simulink model "ShipMPC"  (R2020a)
settings: Solver=VariableStepAuto  StartTime=0.0  StopTime=100  RelTol=1e-3
values from neighbouring files (symbols this model uses):
  tau_wave_amp = 0    [MPCobject.m]
  tau_wave_freq = 0    [MPCobject.m]
  Vc = 0    [MPCobject.m]
  Vref = 0.1    [MPCobject.m]
libraries: mpclib x1
settings Model: Creator=ahaseltalab  LastModifiedBy=localadmin
settings DataIOCC: ReturnWorkspaceOutputs=off
settings DebuggingCC: ArithmeticOperatorsInVariantConditions=warning
settings SFSimCC: SimUseLocalCustomCode=off  CustomCodeUndefinedFunction=UseInterfaceOnly
settings RTWCC: RTWUseLocalCustomCode=off
settings CodeAppCC: StateflowObjectComments=on

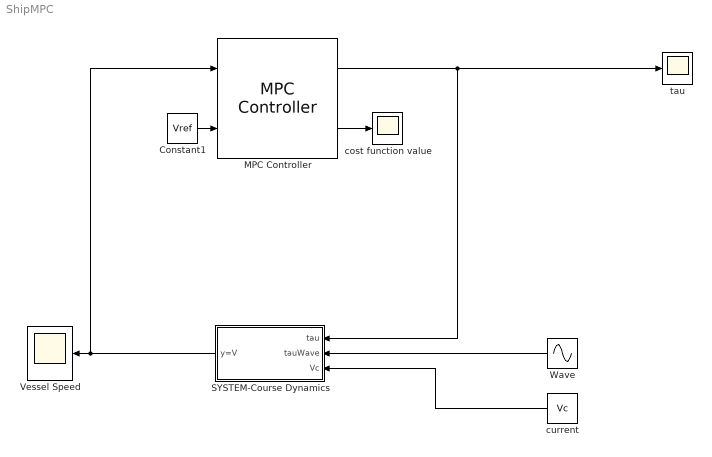
== system ShipMPC ==
  " Wave" : Sin  Amplitude=tau_wave_amp  Frequency=tau_wave_freq  SampleTime=0
  Constant1 : Constant  Value=Vref
  MPC Controller : mpclib/MPC Controller  SCDEnableBlockLinearizationSpecification=on  mpcobj=MPCobj  is_multiple=0  enable_value=0  return_u0=off  updateMPCinCallerWorkspace=on  md_inport=off  mv_inport=off  uref_inport=off  return_cost=on  return_mvseq=off  return_qpstatus=off  return_xseq=off  return_state=off  return_ovseq=off  state_inport=off  umin_inport=off  umax_inport=off  ymin_inport=off  ymax_inport=off  cc_inport=off  ywt_inport=off  uwt_inport=off  duwt_inport=off  rhoeps_inport=off  pm_inport=off  MaximumP=10  HorizonChoice=FixedHorizon  n_ts=1  n_p=20  n_mv=1  n_md=0  n_ud=0  n_mo=1  n_uo=0  BlockDataType=double  SampleTimeInherited=off  switch_inport=off
  SYSTEM-Course Dynamics : Subsystem
  Vessel Speed : Scope
  cost function value : Scope
  current : Constant  Value=Vc
  tau : Scope
  wires:
  MPC Controller/1 -> tau/1, SYSTEM-Course Dynamics/1(tau)
  MPC Controller/2 -> cost function value/1
  Constant1/1 -> MPC Controller/2
  SYSTEM-Course Dynamics/1(y=V) -> MPC Controller/1, Vessel Speed/1
  " Wave"/1 -> SYSTEM-Course Dynamics/2(tauWave)
  current/1 -> SYSTEM-Course Dynamics/3(Vc)

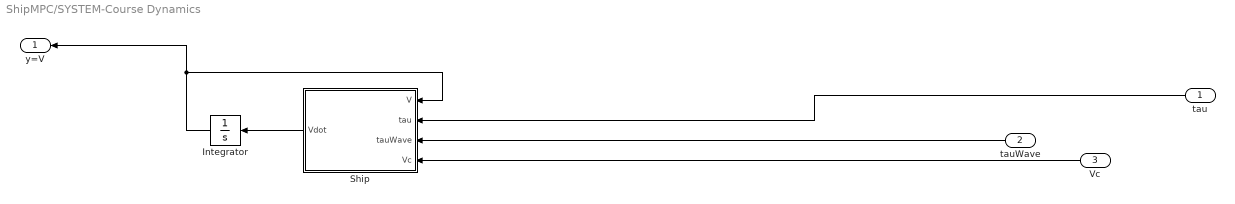
== system ShipMPC/SYSTEM-Course Dynamics ==
  tau : Inport
  tauWave : Inport  Port=2
  Vc : Inport  Port=3
  Integrator : Integrator
  Ship : MATLAB Function  TreatAsAtomicUnit=on
  y=V : Outport
  wires:
  Vc/1 -> Ship/4(Vc)
  tauWave/1 -> Ship/3(tauWave)
  tau/1 -> Ship/2(tau)
  Ship/1(Vdot) -> Integrator/1
  Integrator/1 -> y=V/1, Ship/1(V)

== matlab function ShipMPC/SYSTEM-Course Dynamics/Ship ==
  data: V input; Vdot output; tau input; tauWave input; Vc input
function Vdot = fcn(V,tau,tauWave,Vc)

m=23.8;
ma=2;

Rs=-1.44;


Vdot = (1/(m+ma))*(Rs*(V-Vc)+tau+tauWave);
